simulink model "battery_energy_storage_system"  (R2021a)
settings: Solver=FixedStepDiscrete  StartTime=0.0  StopTime=3  FixedStep=1  RelTol=1e-3
undefined symbols (not defined in the file): CONST
settings Model: Creator=user  LastModifiedBy=user
settings DataIOCC: SaveOutput=off  SignalLogging=off  DSMLogging=off  SaveTime=off  ReturnWorkspaceOutputs=off

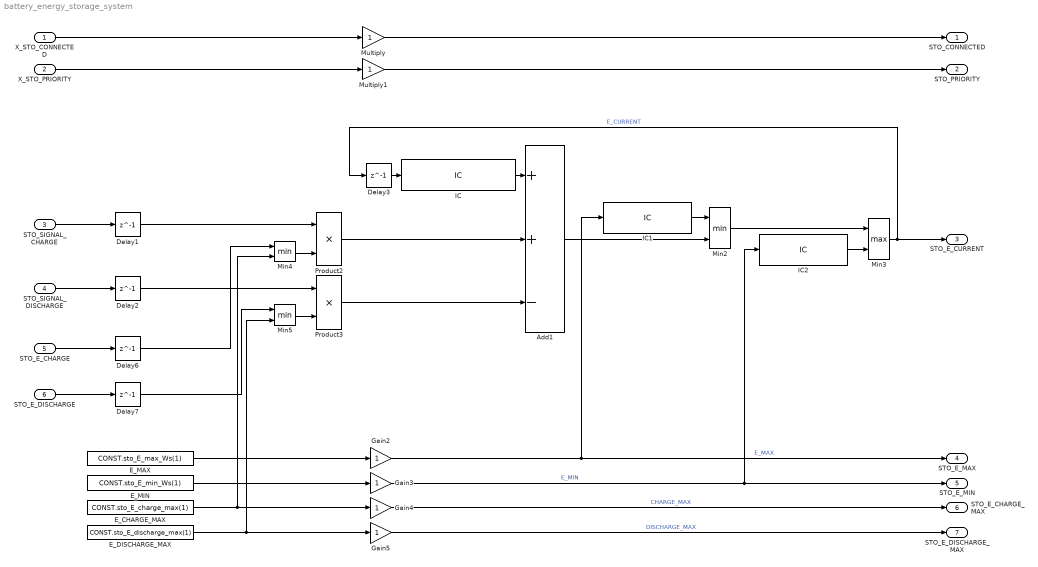
== system battery_energy_storage_system ==
  X_STO_CONNECTED : Inport
  X_STO_PRIORITY : Inport  Port=2
  STO_SIGNAL_CHARGE : Inport  Port=3
  STO_SIGNAL_DISCHARGE : Inport  Port=4
  STO_E_CHARGE : Inport  Port=5
  STO_E_DISCHARGE : Inport  Port=6
  Add1 : Sum  Inputs=++-  InputSameDT=on  OutDataTypeStr=double
  Delay{1..3,6..7} (5 alike) : Delay  DelayLength=1  SampleTime=1
  E_CHARGE_MAX : Constant  Value=CONST.sto_E_charge_max(1)
  E_DISCHARGE_MAX : Constant  Value=CONST.sto_E_discharge_max(1)
  E_MAX : Constant  Value=CONST.sto_E_max_Ws(1)  VectorParams1D=off
  E_MIN : Constant  Value=CONST.sto_E_min_Ws(1)
  Gain{2..5} (4 alike) : Gain
  IC : InitialCondition  Value=CONST.sto_E_current_initial_Ws(1)
  IC1 : InitialCondition  Value=CONST.sto_E_max_Ws(1)
  IC2 : InitialCondition  Value=CONST.sto_E_min_Ws(1)
  Min2 : MinMax  Inputs=2
  Min3 : MinMax  Function=max  Inputs=2
  Min4 : MinMax  Inputs=2
  Min5 : MinMax  Inputs=2
  Multiply : Gain
  Multiply1 : Gain
  Product2 : Product  InputSameDT=on  OutDataTypeStr=double
  Product3 : Product  InputSameDT=on  OutDataTypeStr=double
  STO_CONNECTED : Outport
  STO_PRIORITY : Outport  Port=2
  STO_E_CURRENT : Outport  Port=3
  STO_E_MAX : Outport  Port=4
  STO_E_MIN : Outport  Port=5
  STO_E_CHARGE_MAX : Outport  Port=6
  STO_E_DISCHARGE_MAX : Outport  Port=7
  wires:
  X_STO_CONNECTED/1 -> Multiply/1
  X_STO_PRIORITY/1 -> Multiply1/1
  Gain4/1 -> STO_E_CHARGE_MAX/1  "CHARGE_MAX"
  Min5/1 -> Product3/2
  Gain5/1 -> STO_E_DISCHARGE_MAX/1  "DISCHARGE_MAX"
  E_MAX/1 -> Gain2/1
  Min4/1 -> Product2/2
  E_DISCHARGE_MAX/1 -> Min5/2, Gain5/1
  STO_SIGNAL_CHARGE/1 -> Delay1/1
  Add1/1 -> Min2/2
  Min2/1 -> Min3/1
  STO_E_CHARGE/1 -> Delay6/1
  STO_SIGNAL_DISCHARGE/1 -> Delay2/1
  IC2/1 -> Min3/2
  IC1/1 -> Min2/1
  Gain2/1 -> STO_E_MAX/1, IC1/1  "E_MAX"
  Min3/1 -> STO_E_CURRENT/1, Delay3/1  "E_CURRENT"
  Delay3/1 -> IC/1
  Product3/1 -> Add1/3
  IC/1 -> Add1/1
  E_CHARGE_MAX/1 -> Min4/2, Gain4/1
  Product2/1 -> Add1/2
  E_MIN/1 -> Gain3/1
  Gain3/1 -> STO_E_MIN/1, IC2/1  "E_MIN"
  Multiply/1 -> STO_CONNECTED/1
  Multiply1/1 -> STO_PRIORITY/1
  STO_E_DISCHARGE/1 -> Delay7/1
  Delay1/1 -> Product2/1
  Delay2/1 -> Product3/1
  Delay6/1 -> Min4/1
  Delay7/1 -> Min5/1
